simulink model "Expt3_19EE3FP18"  (R2020b)
settings: Solver=FixedStepAuto  StartTime=0.0  StopTime=10  FixedStep=5e-7  MaxStep=1e-6  RelTol=1e-3
libraries: powerlib x14, simulink x1
settings Model: Creator=swarn  LastModifiedBy=swarn
settings SolverCC: ZeroCrossAlgorithm=Adaptive
settings DebuggingCC: IgnoredZcDiagnostic=none

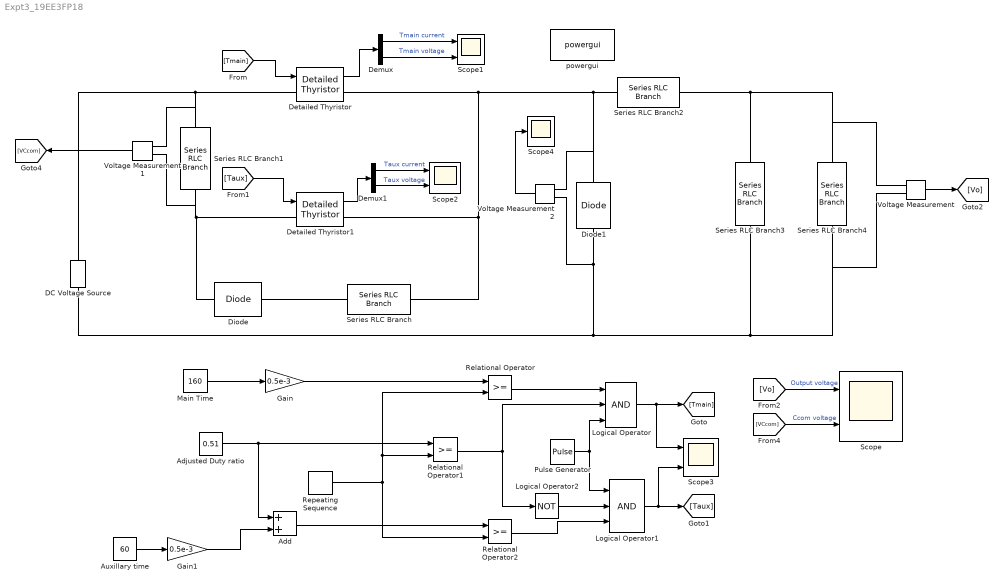
== system Expt3_19EE3FP18 ==
  Add : Sum
  Adjusted Duty ratio : Constant  Value=0.51
  Auxillary time : Constant  Value=60
  DC Voltage Source : powerlib/Electrical Sources/DC Voltage Source  Amplitude=1000  Measurements=None
  Demux : Demux  Outputs=2
      settings: DisplayOption=none
  Demux1 : Demux  Outputs=2
      settings: DisplayOption=none
  Detailed Thyristor : powerlib/Power Electronics/Detailed Thyristor  Ron=1e-6  Lon=1e-3  Vf=0  IL=0.1  Tq=30e-6  IC=0  Rs=inf  Cs=0  Measurements=on
      settings: SourceProductBaseCode=PS
  Detailed Thyristor1 : powerlib/Power Electronics/Detailed Thyristor  Ron=1e-6  Lon=1e-3  Vf=0  IL=0.1  Tq=30e-6  IC=0  Rs=inf  Cs=0  Measurements=on
      settings: SourceProductBaseCode=PS
  Diode : powerlib/Power Electronics/Diode  Ron=1e-6  Lon=0  Vf=0  IC=0  UseSnubber=0  Rs=500  Cs=250e-9  Measurements=off
  Diode1 : powerlib/Power Electronics/Diode  Ron=1e-6  Lon=0  Vf=0  IC=0  UseSnubber=0  Rs=500  Cs=250e-9  Measurements=off
  Gain : Gain  Gain=0.5e-3
  Gain1 : Gain  Gain=0.5e-3
  Logical Operator : Logic  Inputs=3  AllPortsSameDT=off  OutDataTypeStr=boolean
  Logical Operator1 : Logic  Inputs=3  AllPortsSameDT=off  OutDataTypeStr=boolean
  Logical Operator2 : Logic  Operator=NOT  AllPortsSameDT=off  OutDataTypeStr=boolean
  Main Time : Constant  Value=160
  Pulse Generator : DiscretePulseGenerator  PulseType=Time based  Period=20e-6  PulseWidth=50
  Relational Operator : RelationalOperator  OutDataTypeStr=boolean  RndMeth=Simplest
  Relational Operator1 : RelationalOperator  OutDataTypeStr=boolean  RndMeth=Simplest
  Relational Operator2 : RelationalOperator  OutDataTypeStr=boolean  RndMeth=Simplest
  Repeating Sequence : simulink/Sources/Repeating Sequence  rep_seq_t=[0 1]/500  rep_seq_y=[0 1]
  Scope{,1..3} (4 alike) : Scope  NumInputPorts=2
  Scope4 : Scope
  Series RLC Branch : powerlib/Elements/Series RLC Branch  LConnTagsString=__new0  RConnTagsString=__new0  BranchType=L  Resistance=1  Inductance=255e-6  SetiL0=off  InitialCurrent=0  Capacitance=1e-6  Setx0=off  InitialVoltage=0  Measurements=None
  Series RLC Branch1 : powerlib/Elements/Series RLC Branch  LConnTagsString=__new0  RConnTagsString=__new0  BranchType=C  Resistance=1  Inductance=1e-3  SetiL0=off  InitialCurrent=0  Capacitance=3e-6  Setx0=on  InitialVoltage=1000  Measurements=None
  Series RLC Branch2 : powerlib/Elements/Series RLC Branch  LConnTagsString=__new0  RConnTagsString=__new0  BranchType=L  Resistance=1  Inductance=24e-3  SetiL0=off  InitialCurrent=0  Capacitance=1e-6  Setx0=off  InitialVoltage=0  Measurements=None
  Series RLC Branch3 : powerlib/Elements/Series RLC Branch  LConnTagsString=__new0  RConnTagsString=__new0  BranchType=C  Resistance=1  Inductance=1e-3  SetiL0=off  InitialCurrent=0  Capacitance=330e-6  Setx0=off  InitialVoltage=0  Measurements=None
  Series RLC Branch4 : powerlib/Elements/Series RLC Branch  LConnTagsString=__new0  RConnTagsString=__new0  BranchType=R  Resistance=30  Inductance=1e-3  SetiL0=off  InitialCurrent=0  Capacitance=1e-6  Setx0=off  InitialVoltage=0  Measurements=None
  Voltage Measurement : powerlib/Measurements/Voltage Measurement  PhasorSimulation=off  OutputType=Complex  PSBequivalent=0
  Voltage Measurement1 : powerlib/Measurements/Voltage Measurement  PhasorSimulation=off  OutputType=Complex  PSBequivalent=0
  Voltage Measurement2 : powerlib/Measurements/Voltage Measurement  PhasorSimulation=off  OutputType=Complex  PSBequivalent=0
  powergui : powerlib/powergui  Priority=1  SimulationMode=Discrete  SampleTime=5e-7  frequency=60  Iterations=50  frequencyindice=0  Pbase=100e6  ErrMax=1e-4  UnitsV=kV  UnitsW=MW  buscounter=0  FunctionMessages=off  echomessages=off  EnableUseOfTLC=off  CurrentSourceSwitches=off  DisableSnubberDevices=off  DisableRonSwitches=off  DisableVfSwitches=off  DisplayEquations=off  AutomaticDiscreteSolvers=off  SolverType=Tustin/Backward Euler (TBE)  Interpol=off  ExternalGateDelay=off  methode=off  Ts=100  x0status=blocks  SPID=on  SwTol=0  HookPort=off  NonlinearTolerance=1e-4  nMaxIteration=100  ContinueOnMaxIteration=off  RestoreLinks=warning  ResistiveCurrentMeasurement=off  Frange=[0:2:500]  Ylog=off  Xlog=on  ShowGrid=off  save=off  variable=ZData  structure=0  ZoomFFT=off  StartTime=0.0  cycles=1  DisplayStyle=1  fundamental=60  FreqAxis=off  MaxFrequency=1000  frequencyindicesteady=1  RmsSteady=1  display=off
  wires:
  [Tmain] -> Detailed Thyristor/1
  [Taux] -> Detailed Thyristor1/1
  Voltage Measurement/1 -> [Vo]
  [Vo] -> Scope/1  "Output voltage"
  Voltage Measurement1/1 -> [VCcom]
  Detailed Thyristor/1 -> Demux/1
  [VCcom] -> Scope/2  "Ccom voltage"
  Demux/1 -> Scope1/1  "Tmain current"
  Demux/2 -> Scope1/2  "Tmain voltage"
  Demux1/1 -> Scope2/1  "Taux current"
  Demux1/2 -> Scope2/2  "Taux voltage"
  Detailed Thyristor1/1 -> Demux1/1
  Voltage Measurement2/1 -> Scope4/1
  Main Time/1 -> Gain/1
  Gain/1 -> Relational Operator/1
  Relational Operator/1 -> Logical Operator/1
  Relational Operator2/1 -> Logical Operator1/3
  Repeating Sequence/1 -> Relational Operator2/2, Relational Operator/2, Relational Operator1/2
  Adjusted Duty ratio/1 -> Add/1, Relational Operator1/1
  Gain1/1 -> Add/2
  Auxillary time/1 -> Gain1/1
  Add/1 -> Relational Operator2/1
  Relational Operator1/1 -> Logical Operator/2, Logical Operator2/1
  Pulse Generator/1 -> Logical Operator1/1, Logical Operator/3
  Logical Operator/1 -> Scope3/1, [Tmain]
  Logical Operator1/1 -> Scope3/2, [Taux]
  Logical Operator2/1 -> Logical Operator1/2
  connections:
  Diode/LConn1 -- Series RLC Branch/RConn1
  Diode/RConn1 -- Voltage Measurement1/LConn2 -- Series RLC Branch1/RConn1 -- Detailed Thyristor1/LConn1
  Detailed Thyristor1/RConn1 -- Voltage Measurement2/LConn2 -- Diode1/RConn1 -- Series RLC Branch2/LConn1 -- Detailed Thyristor/RConn1 -- Series RLC Branch/LConn1
  DC Voltage Source/RConn1 -- Voltage Measurement1/LConn1 -- Series RLC Branch1/LConn1 -- Detailed Thyristor/LConn1
  Diode1/LConn1 -- Voltage Measurement2/LConn1 -- Voltage Measurement/LConn2 -- Series RLC Branch4/RConn1 -- Series RLC Branch3/RConn1 -- DC Voltage Source/LConn1
  Voltage Measurement/LConn1 -- Series RLC Branch4/LConn1 -- Series RLC Branch2/RConn1 -- Series RLC Branch3/LConn1
